simulink model "controller_archive2"  (R2022b)
settings: Solver=ode4  StartTime=0.0  StopTime=4  FixedStep=0.001  RelTol=1e-3
PreLoadFcn:
  | global m1 m2 l g m1_hat m2_hat;
  | m1 = 2;
  | m2 = 2;
  | m1_hat = 0.97*m1;
  | m2_hat = 0.97*m2;
  | l = 1;
  | g = 9.81;
  | 
  | kd = 200;
  | md = m1_hat;
  | dd = 2*0.7*sqrt(kd*md);
  | 
  | Kd = [kd,0;0,kd];
  | Md = [md,0;0,md];
  | Dd = [dd,0;0,dd];
  | 
  | p = 10^6;
  | d = 2*0.7*sqrt(p);
  | 
  | P = [p,0;0,p];
  | D = [d,0;0,d];
  | 
  | D_hold = D;
  | P_hold = P;
  | 
  | ke = 300;
  | Ke = [ke,0;0,0];
  | 
  | Fc = 1;
  | cv = 4;
  | 
  | delta = 0.01;
  | 
  | x0 = [0.95,0.95];
  | dx0 = [0;0];
  | 
  | n_pow = 0.001;
  | 
  | wall = 0.8;
  | 
  | delay = 2;
libraries: simulink x18, bbblueBasicLib x7
(part 2 of 2)

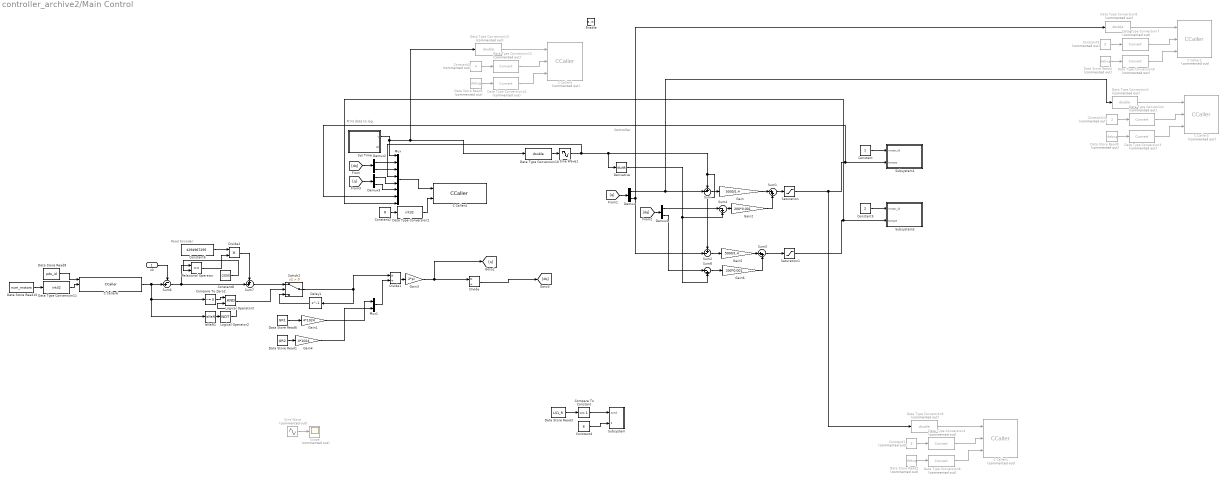
== system controller_archive2/Main Control ==
  note: Controller
  note: Print data to log
  note: Read Encoder
  x0 : Inport
  Enable : EnablePort
  C Caller1 : CCaller  Commented=on  FunctionName=print_input  PortSpecificationStruct="%)30     .    : 4   8    (     @         %    \"     ,    !     0         %  0 \"0    $    _    07)G3F%M90  4&]R=$YA;64 4V-O<&4     26YD97@     5'EP90      4VEZ90      27-';&]B86P   X    P    !@    @    $          4    (     0    $    !         !   0!A    #@   #     &    \"     0         !0    @    !     0    $         $  ! &$    .    .     8    (    !          %    \"     $    %     0         0    !0   $EN<'5T    #@   #@    &    \"     8         !0    @    !     0    $         \"0    @               X    X    !@    @    $          4    (     0    8    !         !     &    9&]U8FQE   .    ,     8    (    !          %    \"     $    !     0         0  $ ,0    X    P    !@    @    ) @        4    (     0    $    !          (  0      #@   #     &    \"     0         !0    @    !     @    $         $  \" &ED   .    ,     8    (    !          %    \"     $    \"     0         0  ( :60   X    X    !@    @    $          4    (     0    4    !         !     %    26YP=70    .    .     8    (    !@         %    \"     $    !     0         )    \"            / _#@   #@    &    \"     0         !0    @    !    !0    $         $     4   !I;G0S,@    X    P    !@    @    $          4    (     0    $    !         !   0 Q    #@   #     &    \"     D\"        !0    @    !     0    $          @ !       .    .     8    (    !          %    \"     $    %     0         0    !0   &1E8G5G    #@   #@    &    \"     0         !0    @    !    !0    $         $     4   !D96)U9P    X    X    !@    @    $          4    (     0    4    !         !     %    26YP=70    .    .     8    (    !@         %    \"     $    !     0         )    \"             ! #@   #@    &    \"     0         !0    @    !    !0    $         $     4   !I;G0S,@    X    P    !@    @    $          4    (     0    $    !         !   0 Q    #@   #     &    \"     D\"        !0    @    !     0    $          @ !"  SampleTime=0.001
  C Caller2 : CCaller  Commented=on  FunctionName=print_input  PortSpecificationStruct="%)30     .    : 4   8    (     @         %    \"     ,    !     0         %  0 \"0    $    _    07)G3F%M90  4&]R=$YA;64 4V-O<&4     26YD97@     5'EP90      4VEZ90      27-';&]B86P   X    P    !@    @    $          4    (     0    $    !         !   0!A    #@   #     &    \"     0         !0    @    !     0    $         $  ! &$    .    .     8    (    !          %    \"     $    %     0         0    !0   $EN<'5T    #@   #@    &    \"     8         !0    @    !     0    $         \"0    @               X    X    !@    @    $          4    (     0    8    !         !     &    9&]U8FQE   .    ,     8    (    !          %    \"     $    !     0         0  $ ,0    X    P    !@    @    ) @        4    (     0    $    !          (  0      #@   #     &    \"     0         !0    @    !     @    $         $  \" &ED   .    ,     8    (    !          %    \"     $    \"     0         0  ( :60   X    X    !@    @    $          4    (     0    4    !         !     %    26YP=70    .    .     8    (    !@         %    \"     $    !     0         )    \"            / _#@   #@    &    \"     0         !0    @    !    !0    $         $     4   !I;G0S,@    X    P    !@    @    $          4    (     0    $    !         !   0 Q    #@   #     &    \"     D\"        !0    @    !     0    $          @ !       .    .     8    (    !          %    \"     $    %     0         0    !0   &1E8G5G    #@   #@    &    \"     0         !0    @    !    !0    $         $     4   !D96)U9P    X    X    !@    @    $          4    (     0    4    !         !     %    26YP=70    .    .     8    (    !@         %    \"     $    !     0         )    \"             ! #@   #@    &    \"     0         !0    @    !    !0    $         $     4   !I;G0S,@    X    P    !@    @    $          4    (     0    $    !         !   0 Q    #@   #     &    \"     D\"        !0    @    !     0    $          @ !"  SampleTime=0.01
  C Caller3 : CCaller  Commented=on  FunctionName=print_input  PortSpecificationStruct="%)30     .    : 4   8    (     @         %    \"     ,    !     0         %  0 \"0    $    _    07)G3F%M90  4&]R=$YA;64 4V-O<&4     26YD97@     5'EP90      4VEZ90      27-';&]B86P   X    P    !@    @    $          4    (     0    $    !         !   0!A    #@   #     &    \"     0         !0    @    !     0    $         $  ! &$    .    .     8    (    !          %    \"     $    %     0         0    !0   $EN<'5T    #@   #@    &    \"     8         !0    @    !     0    $         \"0    @               X    X    !@    @    $          4    (     0    8    !         !     &    9&]U8FQE   .    ,     8    (    !          %    \"     $    !     0         0  $ ,0    X    P    !@    @    ) @        4    (     0    $    !          (  0      #@   #     &    \"     0         !0    @    !     @    $         $  \" &ED   .    ,     8    (    !          %    \"     $    \"     0         0  ( :60   X    X    !@    @    $          4    (     0    4    !         !     %    26YP=70    .    .     8    (    !@         %    \"     $    !     0         )    \"            / _#@   #@    &    \"     0         !0    @    !    !0    $         $     4   !I;G0S,@    X    P    !@    @    $          4    (     0    $    !         !   0 Q    #@   #     &    \"     D\"        !0    @    !     0    $          @ !       .    .     8    (    !          %    \"     $    %     0         0    !0   &1E8G5G    #@   #@    &    \"     0         !0    @    !    !0    $         $     4   !D96)U9P    X    X    !@    @    $          4    (     0    4    !         !     %    26YP=70    .    .     8    (    !@         %    \"     $    !     0         )    \"             ! #@   #@    &    \"     0         !0    @    !    !0    $         $     4   !I;G0S,@    X    P    !@    @    $          4    (     0    $    !         !   0 Q    #@   #     &    \"     D\"        !0    @    !     0    $          @ !"  SampleTime=0.001
  C Caller4 : CCaller  FunctionName=print_data  PortSpecificationStruct="%)30     .    P ,   8    (     @         %    \"     (    !     0         %  0 \"0    $    _    07)G3F%M90  4&]R=$YA;64 4V-O<&4     26YD97@     5'EP90      4VEZ90      27-';&]B86P   X    P    !@    @    $          4    (     0    0    !         !  ! !D871A#@   #     &    \"     0         !0    @    !    !     $         $  $ &1A=&$.    0     8    (    !          %    \"     $    +     0         0    \"P   $EN<'5T3W5T<'5T       .    .     8    (    !@         %    \"     $    !     0         )    \"               #@   #@    &    \"     0         !0    @    !    !@    $         $     8   !D;W5B;&4   X    P    !@    @    $          4    (     0    (    !         !   @ M,0  #@   #     &    \"     D\"        !0    @    !     0    $          @ !       .    ,     8    (    !          %    \"     $    $     0         0  0 <VEZ90X    P    !@    @    $          4    (     0    0    !         !  ! !S:7IE#@   #@    &    \"     0         !0    @    !    !0    $         $     4   !);G!U=     X    X    !@    @    &          4    (     0    $    !          D    (            \\#\\.    .     8    (    !          %    \"     $    %     0         0    !0   &EN=#,R    #@   #     &    \"     0         !0    @    !     0    $         $  ! #$    .    ,     8    (    \"0(        %    \"     $    !     0         \"  $"  SampleTime=0.001
  C Caller5 : CCaller  Commented=on  FunctionName=print_input  PortSpecificationStruct="%)30     .    : 4   8    (     @         %    \"     ,    !     0         %  0 \"0    $    _    07)G3F%M90  4&]R=$YA;64 4V-O<&4     26YD97@     5'EP90      4VEZ90      27-';&]B86P   X    P    !@    @    $          4    (     0    $    !         !   0!A    #@   #     &    \"     0         !0    @    !     0    $         $  ! &$    .    .     8    (    !          %    \"     $    %     0         0    !0   $EN<'5T    #@   #@    &    \"     8         !0    @    !     0    $         \"0    @               X    X    !@    @    $          4    (     0    8    !         !     &    9&]U8FQE   .    ,     8    (    !          %    \"     $    !     0         0  $ ,0    X    P    !@    @    ) @        4    (     0    $    !          (  0      #@   #     &    \"     0         !0    @    !     @    $         $  \" &ED   .    ,     8    (    !          %    \"     $    \"     0         0  ( :60   X    X    !@    @    $          4    (     0    4    !         !     %    26YP=70    .    .     8    (    !@         %    \"     $    !     0         )    \"            / _#@   #@    &    \"     0         !0    @    !    !0    $         $     4   !I;G0S,@    X    P    !@    @    $          4    (     0    $    !         !   0 Q    #@   #     &    \"     D\"        !0    @    !     0    $          @ !       .    .     8    (    !          %    \"     $    %     0         0    !0   &1E8G5G    #@   #@    &    \"     0         !0    @    !    !0    $         $     4   !D96)U9P    X    X    !@    @    $          4    (     0    4    !         !     %    26YP=70    .    .     8    (    !@         %    \"     $    !     0         )    \"             ! #@   #@    &    \"     0         !0    @    !    !0    $         $     4   !I;G0S,@    X    P    !@    @    $          4    (     0    $    !         !   0 Q    #@   #     &    \"     D\"        !0    @    !     0    $          @ !"  SampleTime=0.01
  C Caller6 : CCaller  FunctionName=get_encoder  PortSpecificationStruct="%)30     .    < 4   8    (     @         %    \"     ,    !     0         %  0 \"0    $    _    07)G3F%M90  4&]R=$YA;64 4V-O<&4     26YD97@     5'EP90      4VEZ90      27-';&]B86P   X    X    !@    @    $          4    (     0    8    !         !     &    <&1O7VED   .    .     8    (    !          %    \"     $    &     0         0    !@   '!D;U]I9   #@   #@    &    \"     0         !0    @    !    !0    $         $     4   !);G!U=     X    X    !@    @    &          4    (     0    $    !          D    (               .    .     8    (    !          %    \"     $    %     0         0    !0   &EN=#,R    #@   #     &    \"     0         !0    @    !     0    $         $  ! #$    .    ,     8    (    \"0(        %    \"     $    !     0         \"  $       X    P    !@    @    $          4    (     0    0    !         !  ! !S:7IE#@   #     &    \"     0         !0    @    !    !     $         $  $ '-I>F4.    .     8    (    !          %    \"     $    %     0         0    !0   $EN<'5T    #@   #@    &    \"     8         !0    @    !     0    $         \"0    @           #P/PX    X    !@    @    $          4    (     0    4    !         !     %    :6YT,S(    .    ,     8    (    !          %    \"     $    !     0         0  $ ,0    X    P    !@    @    ) @        4    (     0    $    !          (  0      #@   #     &    \"     0         !0    @    !     P    $         $  # '!O<P .    ,     8    (    !          %    \"     $    #     0         0  , <&]S  X   !     !@    @    $          4    (     0    L    !         !     +    26YP=71/=71P=70       X    X    !@    @    &          4    (     0    $    !          D    (             $ .    .     8    (    !          %    \"     $    &     0         0    !@   &1O=6)L90  #@   #     &    \"     0         !0    @    !     0    $         $  ! #(    .    ,     8    (    \"0(        %    \"     $    !     0         \"  $"  SampleTime=0.001
  Compare To Constant : simulink/Logic and Bit Operations/Compare To Constant  relop===  const=1  OutDataTypeStr=boolean
  Compare To Zero2 : simulink/Logic and Bit Operations/Compare To Zero  relop=~=  OutDataTypeStr=boolean
  Constant : Constant
  Constant1 : Constant  Commented=on  Value=3
  Constant14 : Constant  Commented=on  Value=2
  Constant2 : Constant  Value=8
  Constant3 : Constant  Commented=on  Value=4
  Constant4 : Constant  Value=6
  Constant5 : Constant  Value=2
  Constant6 : Constant  Value=4294967295
  Constant8 : Constant  Value=-2000
  Constant9 : Constant  Commented=on  Value=3
  Data Store Read1 : DataStoreRead  DataStoreName=GR2  IndexOptions=Index vector (dialog)  Indices=1  OutputSizes=1
  Data Store Read10 : DataStoreRead  DataStoreName=num_motors  IndexOptions=Index vector (dialog)  Indices=1  OutputSizes=1
  Data Store Read{2,4..5,9} (4 alike) : DataStoreRead  Commented=on  DataStoreName=debug  IndexOptions=Index vector (dialog)  Indices=1  OutputSizes=1
  Data Store Read3 : DataStoreRead  DataStoreName=LS1_R  IndexOptions=Index vector (dialog)  Indices=1  OutputSizes=1
  Data Store Read6 : DataStoreRead  DataStoreName=GR1  IndexOptions=Index vector (dialog)  Indices=1  OutputSizes=1
  Data Store Read8 : DataStoreRead  DataStoreName=pdo_id  IndexOptions=Index vector (dialog)  Indices=1  OutputSizes=1
  Data Type Conversion{,3..4,6..7,9,12,14} (8 alike) : DataTypeConversion  Commented=on  SaturateOnIntegerOverflow=off  RndMeth=Floor
  Data Type Conversion{1,5,8,13} (4 alike) : DataTypeConversion  Commented=on  OutDataTypeStr=double  SaturateOnIntegerOverflow=off  RndMeth=Floor
  Data Type Conversion10 : DataTypeConversion  OutDataTypeStr=double  SaturateOnIntegerOverflow=off  RndMeth=Floor
  Data Type Conversion11 : DataTypeConversion  OutDataTypeStr=int32  SaturateOnIntegerOverflow=off  RndMeth=Floor
  Data Type Conversion2 : DataTypeConversion  OutDataTypeStr=int32  SaturateOnIntegerOverflow=off  RndMeth=Floor
  Delay1 : Delay  DelayLength=1  InitialCondition=0
  Demux{,1..3} (4 alike) : Demux  Outputs=2
  Derivative : Derivative
  Divide : Product  Inputs=*/
  Divide1 : Product  Inputs=*/
  Divide2 : Product  Inputs=**
  Gain : Gain  Gain=5000/1.4
  Gain1 : Gain  Gain=4*1024
  Gain2 : Gain  Gain=200*0.001
  Gain3 : Gain  Gain=2*pi
  Gain4 : Gain  Gain=4*1024
  Gain5 : Gain  Gain=5000/1.4
  Gain6 : Gain  Gain=200*0.001
  IsNaN1 : RelationalOperator  Operator=isNaN  OutDataTypeStr=boolean  RndMeth=Simplest  InputSameDT=off
  Logical Operator2 : Logic  Operator=NOT  AllPortsSameDT=off  OutDataTypeStr=boolean
  Logical Operator3 : Logic  AllPortsSameDT=off  OutDataTypeStr=boolean
  Mux : Mux  Inputs=8
  Mux1 : Mux  Inputs=2
  Relational Operator : RelationalOperator  Operator=<=  OutDataTypeStr=boolean  RndMeth=Simplest  InputSameDT=off
  Saturation : Saturate  UpperLimit=400  LowerLimit=-400
  Saturation1 : Saturate  UpperLimit=400  LowerLimit=-400
  Scope : Scope  Commented=on
  Sine Wave : Sin  Commented=on  Amplitude=0.3  Bias=0.5  Frequency=0.1  SampleTime=0
  Sine Wave1 : Sin  TimeSource=Use external signal  Amplitude=0.3  Bias=0.3  Frequency=1.5  Phase=-pi/2  SampleTime=0
  Subsystem : Subsystem
  Subsystem1 : Subsystem
  Subsystem2 : Subsystem
  Sum : Sum  Inputs=+-|
  Sum1 : Sum  Inputs=|++
  Sum2 : Sum  Inputs=+-|
  Sum3 : Sum  Inputs=|++
  Sum4 : Sum  Inputs=|-+
  Sum6 : Sum  Inputs=-+|
  Sum7 : Sum  Inputs=++|
  Sum8 : Sum  Inputs=|-+
  Switch2 : Switch  Criteria=u2 > Threshold  SaturateOnIntegerOverflow=off  InputSameDT=off
  Sys Time : Subsystem
  wires:
  Constant/1 -> Subsystem1/1(motor_id)
  Constant2/1 -> Data Type Conversion2/1
  Mux/1 -> C Caller4/1
  Sys Time/1(t) -> Mux/1, Data Type Conversion13/1, Data Type Conversion10/1
  Data Type Conversion2/1 -> C Caller4/2
  [dq] -> Demux2/1
  Compare To Constant/1 -> Subsystem/1(cond)
  Constant4/1 -> Subsystem/2(new_state)
  Data Store Read3/1 -> Compare To Constant/1
  Constant14/1 -> Data Type Conversion/1
  Data Type Conversion3/1 -> C Caller3/3
  Data Store Read9/1 -> Data Type Conversion3/1
  Data Type Conversion/1 -> C Caller3/2
  Data Type Conversion1/1 -> C Caller3/1
  Data Store Read10/1 -> Data Type Conversion11/1
  Compare To Zero2/1 -> Logical Operator3/1
  Logical Operator2/1 -> Logical Operator3/2
  Delay1/1 -> Switch2/3
  IsNaN1/1 -> Logical Operator2/1
  Divide1/1 -> Gain3/1
  Logical Operator3/1 -> Switch2/2
  Data Store Read6/1 -> Gain1/1
  Gain1/1 -> Mux1/1
  Gain3/1 -> Divide/1, [q]
  Data Store Read8/1 -> C Caller6/1
  Divide/1 -> [dq]
  Data Type Conversion11/1 -> C Caller6/2
  x0/1 -> Sum6/1
  Sum6/1 -> Relational Operator/1, Sum7/2
  Constant6/1 -> Divide2/1
  Divide2/1 -> Sum7/1
  Sum7/1 -> Switch2/1
  Saturation/1 -> Data Type Conversion5/1, Mux/7, Subsystem1/2(torque)
  Sum/1 -> Gain/1
  Gain/1 -> Sum1/1
  [dq] -> Demux1/1
  Demux1/1 -> Sum4/1
  Sum1/1 -> Saturation/1
  [q] -> Demux/1
  Mux1/1 -> Divide1/2
  Data Store Read1/1 -> Gain4/1
  Gain4/1 -> Mux1/2
  Data Type Conversion5/1 -> C Caller1/1
  Data Type Conversion4/1 -> C Caller1/2
  Constant1/1 -> Data Type Conversion4/1
  Data Store Read2/1 -> Data Type Conversion6/1
  Data Type Conversion6/1 -> C Caller1/3
  Constant5/1 -> Subsystem2/1(motor_id)
  Saturation1/1 -> Mux/8, Subsystem2/2(torque)
  Sum3/1 -> Saturation1/1
  Gain6/1 -> Sum3/2
  Gain5/1 -> Sum3/1
  Demux/2 -> Sum2/2, Data Type Conversion8/1
  Sum2/1 -> Gain5/1
  Switch2/1 -> Divide1/1, Delay1/1
  Relational Operator/1 -> Divide2/2
  Constant8/1 -> Relational Operator/2
  C Caller6/1 -> IsNaN1/1, Compare To Zero2/1, Sum6/2
  Sine Wave/1 -> Scope/1
  Sum4/1 -> Gain2/1
  Sine Wave1/1 -> Mux/4, Sum2/1, Sum/1, Derivative/1
  Data Type Conversion8/1 -> C Caller2/1
  Data Type Conversion7/1 -> C Caller2/2
  Data Store Read4/1 -> Data Type Conversion9/1
  Constant9/1 -> Data Type Conversion7/1
  Data Type Conversion9/1 -> C Caller2/3
  Data Type Conversion10/1 -> Sine Wave1/1
  Gain2/1 -> Sum1/2
  Sum8/1 -> Gain6/1
  Derivative/1 -> Sum8/2, Sum4/2
  Demux1/2 -> Sum8/1
  Demux2/1 -> Mux/2
  Demux2/2 -> Mux/3
  Demux/1 -> Data Type Conversion1/1, Sum/2
  Data Type Conversion14/1 -> C Caller5/3
  Data Store Read5/1 -> Data Type Conversion14/1
  Data Type Conversion12/1 -> C Caller5/2
  Constant3/1 -> Data Type Conversion12/1
  Data Type Conversion13/1 -> C Caller5/1
  Demux3/1 -> Mux/5
  Demux3/2 -> Mux/6
  [q] -> Demux3/1

== system controller_archive2/Home1/Stop Motor1 ==
  Trigger : TriggerPort  VariantControl=(inherit)
  C Caller4 : CCaller  FunctionName=stop_motor  PortSpecificationStruct="%)30     .    Z ,   8    (     @         %    \"     (    !     0         %  0 \"0    $    _    07)G3F%M90  4&]R=$YA;64 4V-O<&4     26YD97@     5'EP90      4VEZ90      27-';&]B86P   X    X    !@    @    $          4    (     0    8    !         !     &    <&1O7V9D   .    .     8    (    !          %    \"     $    &     0         0    !@   '!D;U]F9   #@   #@    &    \"     0         !0    @    !    !0    $         $     4   !);G!U=     X    X    !@    @    &          4    (     0    $    !          D    (               .    .     8    (    !          %    \"     $    %     0         0    !0   &EN=#,R    #@   #     &    \"     0         !0    @    !     0    $         $  ! #$    .    ,     8    (    \"0(        %    \"     $    !     0         \"  $       X   !     !@    @    $          4    (     0    H    !         !     *    ;G5M7VUO=&]R<P        X   !     !@    @    $          4    (     0    H    !         !     *    ;G5M7VUO=&]R<P        X    X    !@    @    $          4    (     0    4    !         !     %    26YP=70    .    .     8    (    !@         %    \"     $    !     0         )    \"            / _#@   #@    &    \"     0         !0    @    !    !0    $         $     4   !I;G0S,@    X    P    !@    @    $          4    (     0    $    !         !   0 Q    #@   #     &    \"     D\"        !0    @    !     0    $          @ !"
  Data Store Read1 : DataStoreRead  DataStoreName=pdo_id  IndexOptions=Index vector (dialog)  Indices=1  OutputSizes=1
  Data Store Read7 : DataStoreRead  DataStoreName=num_motors  IndexOptions=Index vector (dialog)  Indices=1  OutputSizes=1
  Data Type Conversion : DataTypeConversion  OutDataTypeStr=int32  SaturateOnIntegerOverflow=off  RndMeth=Floor
  wires:
  Data Store Read1/1 -> C Caller4/1
  Data Store Read7/1 -> Data Type Conversion/1
  Data Type Conversion/1 -> C Caller4/2

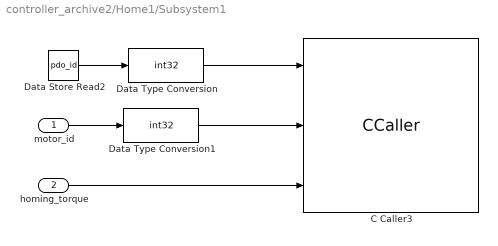
== system controller_archive2/Home1/Subsystem1 ==
  motor_id : Inport
  homing_torque : Inport  Port=2
  C Caller3 : CCaller  FunctionName=set_motor  PortSpecificationStruct="%)30     .    B 4   8    (     @         %    \"     ,    !     0         %  0 \"0    $    _    07)G3F%M90  4&]R=$YA;64 4V-O<&4     26YD97@     5'EP90      4VEZ90      27-';&]B86P   X    X    !@    @    $          4    (     0    8    !         !     &    <&1O7VED   .    .     8    (    !          %    \"     $    &     0         0    !@   '!D;U]I9   #@   #@    &    \"     0         !0    @    !    !0    $         $     4   !);G!U=     X    X    !@    @    &          4    (     0    $    !          D    (               .    .     8    (    !          %    \"     $    %     0         0    !0   &EN=#,R    #@   #     &    \"     0         !0    @    !     0    $         $  ! #$    .    ,     8    (    \"0(        %    \"     $    !     0         \"  $       X    X    !@    @    $          4    (     0    @    !         !     (    ;6]T;W)?:60.    .     8    (    !          %    \"     $    (     0         0    \"    &UO=&]R7VED#@   #@    &    \"     0         !0    @    !    !0    $         $     4   !);G!U=     X    X    !@    @    &          4    (     0    $    !          D    (            \\#\\.    .     8    (    !          %    \"     $    %     0         0    !0   &EN=#,R    #@   #     &    \"     0         !0    @    !     0    $         $  ! #$    .    ,     8    (    \"0(        %    \"     $    !     0         \"  $       X    X    !@    @    $          4    (     0    <    !         !     '    <V5T7W9A;  .    .     8    (    !          %    \"     $    '     0         0    !P   '-E=%]V86P #@   #@    &    \"     0         !0    @    !    !0    $         $     4   !);G!U=     X    X    !@    @    &          4    (     0    $    !          D    (             $ .    .     8    (    !          %    \"     $    &     0         0    !@   &1O=6)L90  #@   #     &    \"     0         !0    @    !     0    $         $  ! #$    .    ,     8    (    \"0(        %    \"     $    !     0         \"  $"  SampleTime=0.001
  Data Store Read2 : DataStoreRead  DataStoreName=pdo_id  IndexOptions=Index vector (dialog)  Indices=1  OutputSizes=1
  Data Type Conversion : DataTypeConversion  OutDataTypeStr=int32  SaturateOnIntegerOverflow=off  RndMeth=Floor
  Data Type Conversion1 : DataTypeConversion  OutDataTypeStr=int32  SaturateOnIntegerOverflow=off  RndMeth=Floor
  wires:
  motor_id/1 -> Data Type Conversion1/1
  Data Store Read2/1 -> Data Type Conversion/1
  Data Type Conversion/1 -> C Caller3/1
  Data Type Conversion1/1 -> C Caller3/2
  homing_torque/1 -> C Caller3/3

== system controller_archive2/Home1/Subsystem2 ==
  cond : Inport
  new_state : Inport  Port=2
  Data Store Read : DataStoreRead  DataStoreName=state  IndexOptions=Index vector (dialog)  Indices=1  OutputSizes=1
  Data Store Write : DataStoreWrite  DataStoreName=state  IndexOptions=Index vector (dialog)  Indices=1  OutputSizes=1
  Switch : Switch  Criteria=u2 > Threshold  SaturateOnIntegerOverflow=off  InputSameDT=off
  wires:
  new_state/1 -> Switch/1
  Data Store Read/1 -> Switch/3
  Switch/1 -> Data Store Write/1
  cond/1 -> Switch/2

== system controller_archive2/Home2/Stop Motor1 ==
  Trigger : TriggerPort  VariantControl=(inherit)
  C Caller4 : CCaller  FunctionName=stop_motor  PortSpecificationStruct="%)30     .    Z ,   8    (     @         %    \"     (    !     0         %  0 \"0    $    _    07)G3F%M90  4&]R=$YA;64 4V-O<&4     26YD97@     5'EP90      4VEZ90      27-';&]B86P   X    X    !@    @    $          4    (     0    8    !         !     &    <&1O7V9D   .    .     8    (    !          %    \"     $    &     0         0    !@   '!D;U]F9   #@   #@    &    \"     0         !0    @    !    !0    $         $     4   !);G!U=     X    X    !@    @    &          4    (     0    $    !          D    (               .    .     8    (    !          %    \"     $    %     0         0    !0   &EN=#,R    #@   #     &    \"     0         !0    @    !     0    $         $  ! #$    .    ,     8    (    \"0(        %    \"     $    !     0         \"  $       X   !     !@    @    $          4    (     0    H    !         !     *    ;G5M7VUO=&]R<P        X   !     !@    @    $          4    (     0    H    !         !     *    ;G5M7VUO=&]R<P        X    X    !@    @    $          4    (     0    4    !         !     %    26YP=70    .    .     8    (    !@         %    \"     $    !     0         )    \"            / _#@   #@    &    \"     0         !0    @    !    !0    $         $     4   !I;G0S,@    X    P    !@    @    $          4    (     0    $    !         !   0 Q    #@   #     &    \"     D\"        !0    @    !     0    $          @ !"
  Data Store Read1 : DataStoreRead  DataStoreName=pdo_id  IndexOptions=Index vector (dialog)  Indices=1  OutputSizes=1
  Data Store Read7 : DataStoreRead  DataStoreName=num_motors  IndexOptions=Index vector (dialog)  Indices=1  OutputSizes=1
  Data Type Conversion : DataTypeConversion  OutDataTypeStr=int32  SaturateOnIntegerOverflow=off  RndMeth=Floor
  wires:
  Data Store Read1/1 -> C Caller4/1
  Data Store Read7/1 -> Data Type Conversion/1
  Data Type Conversion/1 -> C Caller4/2

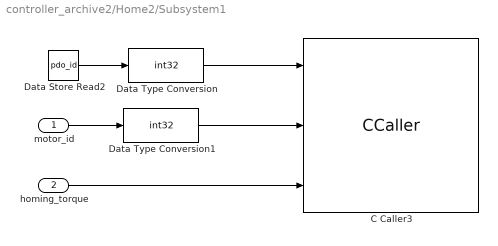
== system controller_archive2/Home2/Subsystem1 ==
  motor_id : Inport
  homing_torque : Inport  Port=2
  C Caller3 : CCaller  FunctionName=set_motor  PortSpecificationStruct="%)30     .    B 4   8    (     @         %    \"     ,    !     0         %  0 \"0    $    _    07)G3F%M90  4&]R=$YA;64 4V-O<&4     26YD97@     5'EP90      4VEZ90      27-';&]B86P   X    X    !@    @    $          4    (     0    8    !         !     &    <&1O7VED   .    .     8    (    !          %    \"     $    &     0         0    !@   '!D;U]I9   #@   #@    &    \"     0         !0    @    !    !0    $         $     4   !);G!U=     X    X    !@    @    &          4    (     0    $    !          D    (               .    .     8    (    !          %    \"     $    %     0         0    !0   &EN=#,R    #@   #     &    \"     0         !0    @    !     0    $         $  ! #$    .    ,     8    (    \"0(        %    \"     $    !     0         \"  $       X    X    !@    @    $          4    (     0    @    !         !     (    ;6]T;W)?:60.    .     8    (    !          %    \"     $    (     0         0    \"    &UO=&]R7VED#@   #@    &    \"     0         !0    @    !    !0    $         $     4   !);G!U=     X    X    !@    @    &          4    (     0    $    !          D    (            \\#\\.    .     8    (    !          %    \"     $    %     0         0    !0   &EN=#,R    #@   #     &    \"     0         !0    @    !     0    $         $  ! #$    .    ,     8    (    \"0(        %    \"     $    !     0         \"  $       X    X    !@    @    $          4    (     0    <    !         !     '    <V5T7W9A;  .    .     8    (    !          %    \"     $    '     0         0    !P   '-E=%]V86P #@   #@    &    \"     0         !0    @    !    !0    $         $     4   !);G!U=     X    X    !@    @    &          4    (     0    $    !          D    (             $ .    .     8    (    !          %    \"     $    &     0         0    !@   &1O=6)L90  #@   #     &    \"     0         !0    @    !     0    $         $  ! #$    .    ,     8    (    \"0(        %    \"     $    !     0         \"  $"  SampleTime=0.001
  Data Store Read2 : DataStoreRead  DataStoreName=pdo_id  IndexOptions=Index vector (dialog)  Indices=1  OutputSizes=1
  Data Type Conversion : DataTypeConversion  OutDataTypeStr=int32  SaturateOnIntegerOverflow=off  RndMeth=Floor
  Data Type Conversion1 : DataTypeConversion  OutDataTypeStr=int32  SaturateOnIntegerOverflow=off  RndMeth=Floor
  wires:
  motor_id/1 -> Data Type Conversion1/1
  Data Store Read2/1 -> Data Type Conversion/1
  Data Type Conversion/1 -> C Caller3/1
  Data Type Conversion1/1 -> C Caller3/2
  homing_torque/1 -> C Caller3/3

== system controller_archive2/Home2/Subsystem2 ==
  cond : Inport
  new_state : Inport  Port=2
  Data Store Read : DataStoreRead  DataStoreName=state  IndexOptions=Index vector (dialog)  Indices=1  OutputSizes=1
  Data Store Write : DataStoreWrite  DataStoreName=state  IndexOptions=Index vector (dialog)  Indices=1  OutputSizes=1
  Switch : Switch  Criteria=u2 > Threshold  SaturateOnIntegerOverflow=off  InputSameDT=off
  wires:
  new_state/1 -> Switch/1
  Data Store Read/1 -> Switch/3
  Switch/1 -> Data Store Write/1
  cond/1 -> Switch/2

== system controller_archive2/Home3/Stop Motor1 ==
  Trigger : TriggerPort  VariantControl=(inherit)
  C Caller4 : CCaller  FunctionName=stop_motor
  Data Store Read1 : DataStoreRead  DataStoreName=pdo_id  IndexOptions=Index vector (dialog)  Indices=1  OutputSizes=1
  Data Store Read7 : DataStoreRead  DataStoreName=num_motors  IndexOptions=Index vector (dialog)  Indices=1  OutputSizes=1
  Data Type Conversion : DataTypeConversion  OutDataTypeStr=int32  SaturateOnIntegerOverflow=off  RndMeth=Floor
  wires:
  Data Store Read1/1 -> C Caller4/1
  Data Store Read7/1 -> Data Type Conversion/1
  Data Type Conversion/1 -> C Caller4/2

== system controller_archive2/Home3/Subsystem1 ==
  motor_id : Inport
  homing_torque : Inport  Port=2
  C Caller3 : CCaller  FunctionName=set_motor  SampleTime=0.001
  Data Store Read2 : DataStoreRead  DataStoreName=pdo_id  IndexOptions=Index vector (dialog)  Indices=1  OutputSizes=1
  Data Type Conversion : DataTypeConversion  OutDataTypeStr=int32  SaturateOnIntegerOverflow=off  RndMeth=Floor
  Data Type Conversion1 : DataTypeConversion  OutDataTypeStr=int32  SaturateOnIntegerOverflow=off  RndMeth=Floor
  wires:
  motor_id/1 -> Data Type Conversion1/1
  Data Store Read2/1 -> Data Type Conversion/1
  Data Type Conversion/1 -> C Caller3/1
  Data Type Conversion1/1 -> C Caller3/2
  homing_torque/1 -> C Caller3/3

== system controller_archive2/Home3/Subsystem2 ==
  cond : Inport
  new_state : Inport  Port=2
  Data Store Read : DataStoreRead  DataStoreName=state  IndexOptions=Index vector (dialog)  Indices=1  OutputSizes=1
  Data Store Write : DataStoreWrite  DataStoreName=state  IndexOptions=Index vector (dialog)  Indices=1  OutputSizes=1
  Switch : Switch  Criteria=u2 > Threshold  SaturateOnIntegerOverflow=off  InputSameDT=off
  wires:
  new_state/1 -> Switch/1
  Data Store Read/1 -> Switch/3
  Switch/1 -> Data Store Write/1
  cond/1 -> Switch/2

== system controller_archive2/Home4/Stop Motor1 ==
  Trigger : TriggerPort  VariantControl=(inherit)
  C Caller4 : CCaller  FunctionName=stop_motor
  Data Store Read1 : DataStoreRead  DataStoreName=pdo_id  IndexOptions=Index vector (dialog)  Indices=1  OutputSizes=1
  Data Store Read7 : DataStoreRead  DataStoreName=num_motors  IndexOptions=Index vector (dialog)  Indices=1  OutputSizes=1
  Data Type Conversion : DataTypeConversion  OutDataTypeStr=int32  SaturateOnIntegerOverflow=off  RndMeth=Floor
  wires:
  Data Store Read1/1 -> C Caller4/1
  Data Store Read7/1 -> Data Type Conversion/1
  Data Type Conversion/1 -> C Caller4/2

== system controller_archive2/Home4/Subsystem1 ==
  motor_id : Inport
  homing_torque : Inport  Port=2
  C Caller3 : CCaller  FunctionName=set_motor  SampleTime=0.001
  Data Store Read2 : DataStoreRead  DataStoreName=pdo_id  IndexOptions=Index vector (dialog)  Indices=1  OutputSizes=1
  Data Type Conversion : DataTypeConversion  OutDataTypeStr=int32  SaturateOnIntegerOverflow=off  RndMeth=Floor
  Data Type Conversion1 : DataTypeConversion  OutDataTypeStr=int32  SaturateOnIntegerOverflow=off  RndMeth=Floor
  wires:
  motor_id/1 -> Data Type Conversion1/1
  Data Store Read2/1 -> Data Type Conversion/1
  Data Type Conversion/1 -> C Caller3/1
  Data Type Conversion1/1 -> C Caller3/2
  homing_torque/1 -> C Caller3/3

== system controller_archive2/Home4/Subsystem2 ==
  cond : Inport
  new_state : Inport  Port=2
  Data Store Read : DataStoreRead  DataStoreName=state  IndexOptions=Index vector (dialog)  Indices=1  OutputSizes=1
  Data Store Write : DataStoreWrite  DataStoreName=state  IndexOptions=Index vector (dialog)  Indices=1  OutputSizes=1
  Switch : Switch  Criteria=u2 > Threshold  SaturateOnIntegerOverflow=off  InputSameDT=off
  wires:
  new_state/1 -> Switch/1
  Data Store Read/1 -> Switch/3
  Switch/1 -> Data Store Write/1
  cond/1 -> Switch/2

== system controller_archive2/Initialize/Subsystem ==
  cond : Inport
  new_state : Inport  Port=2
  Data Store Read : DataStoreRead  DataStoreName=state  IndexOptions=Index vector (dialog)  Indices=1  OutputSizes=1
  Data Store Write : DataStoreWrite  DataStoreName=state  IndexOptions=Index vector (dialog)  Indices=1  OutputSizes=1
  Switch : Switch  Criteria=u2 > Threshold  SaturateOnIntegerOverflow=off  InputSameDT=off
  wires:
  new_state/1 -> Switch/1
  Data Store Read/1 -> Switch/3
  Switch/1 -> Data Store Write/1
  cond/1 -> Switch/2

== system controller_archive2/Main Control/Subsystem ==
  cond : Inport
  new_state : Inport  Port=2
  Data Store Read : DataStoreRead  DataStoreName=state  IndexOptions=Index vector (dialog)  Indices=1  OutputSizes=1
  Data Store Write : DataStoreWrite  DataStoreName=state  IndexOptions=Index vector (dialog)  Indices=1  OutputSizes=1
  Switch : Switch  Criteria=u2 > Threshold  SaturateOnIntegerOverflow=off  InputSameDT=off
  wires:
  new_state/1 -> Switch/1
  Data Store Read/1 -> Switch/3
  Switch/1 -> Data Store Write/1
  cond/1 -> Switch/2

== system controller_archive2/Main Control/Subsystem1 ==
  motor_id : Inport
  torque : Inport  Port=2
  C Caller3 : CCaller  FunctionName=set_motor  PortSpecificationStruct="%)30     .    B 4   8    (     @         %    \"     ,    !     0         %  0 \"0    $    _    07)G3F%M90  4&]R=$YA;64 4V-O<&4     26YD97@     5'EP90      4VEZ90      27-';&]B86P   X    X    !@    @    $          4    (     0    8    !         !     &    <&1O7VED   .    .     8    (    !          %    \"     $    &     0         0    !@   '!D;U]I9   #@   #@    &    \"     0         !0    @    !    !0    $         $     4   !);G!U=     X    X    !@    @    &          4    (     0    $    !          D    (               .    .     8    (    !          %    \"     $    %     0         0    !0   &EN=#,R    #@   #     &    \"     0         !0    @    !     0    $         $  ! #$    .    ,     8    (    \"0(        %    \"     $    !     0         \"  $       X    X    !@    @    $          4    (     0    @    !         !     (    ;6]T;W)?:60.    .     8    (    !          %    \"     $    (     0         0    \"    &UO=&]R7VED#@   #@    &    \"     0         !0    @    !    !0    $         $     4   !);G!U=     X    X    !@    @    &          4    (     0    $    !          D    (            \\#\\.    .     8    (    !          %    \"     $    %     0         0    !0   &EN=#,R    #@   #     &    \"     0         !0    @    !     0    $         $  ! #$    .    ,     8    (    \"0(        %    \"     $    !     0         \"  $       X    X    !@    @    $          4    (     0    <    !         !     '    <V5T7W9A;  .    .     8    (    !          %    \"     $    '     0         0    !P   '-E=%]V86P #@   #@    &    \"     0         !0    @    !    !0    $         $     4   !);G!U=     X    X    !@    @    &          4    (     0    $    !          D    (             $ .    .     8    (    !          %    \"     $    &     0         0    !@   &1O=6)L90  #@   #     &    \"     0         !0    @    !     0    $         $  ! #$    .    ,     8    (    \"0(        %    \"     $    !     0         \"  $"  SampleTime=0.001
  Data Store Read2 : DataStoreRead  DataStoreName=pdo_id  IndexOptions=Index vector (dialog)  Indices=1  OutputSizes=1
  Data Type Conversion : DataTypeConversion  OutDataTypeStr=int32  SaturateOnIntegerOverflow=off  RndMeth=Floor
  Data Type Conversion1 : DataTypeConversion  OutDataTypeStr=int32  SaturateOnIntegerOverflow=off  RndMeth=Floor
  wires:
  motor_id/1 -> Data Type Conversion1/1
  Data Store Read2/1 -> Data Type Conversion/1
  Data Type Conversion/1 -> C Caller3/1
  Data Type Conversion1/1 -> C Caller3/2
  torque/1 -> C Caller3/3

== system controller_archive2/Main Control/Subsystem2 ==
  motor_id : Inport
  torque : Inport  Port=2
  C Caller3 : CCaller  FunctionName=set_motor  PortSpecificationStruct="%)30     .    B 4   8    (     @         %    \"     ,    !     0         %  0 \"0    $    _    07)G3F%M90  4&]R=$YA;64 4V-O<&4     26YD97@     5'EP90      4VEZ90      27-';&]B86P   X    X    !@    @    $          4    (     0    8    !         !     &    <&1O7VED   .    .     8    (    !          %    \"     $    &     0         0    !@   '!D;U]I9   #@   #@    &    \"     0         !0    @    !    !0    $         $     4   !);G!U=     X    X    !@    @    &          4    (     0    $    !          D    (               .    .     8    (    !          %    \"     $    %     0         0    !0   &EN=#,R    #@   #     &    \"     0         !0    @    !     0    $         $  ! #$    .    ,     8    (    \"0(        %    \"     $    !     0         \"  $       X    X    !@    @    $          4    (     0    @    !         !     (    ;6]T;W)?:60.    .     8    (    !          %    \"     $    (     0         0    \"    &UO=&]R7VED#@   #@    &    \"     0         !0    @    !    !0    $         $     4   !);G!U=     X    X    !@    @    &          4    (     0    $    !          D    (            \\#\\.    .     8    (    !          %    \"     $    %     0         0    !0   &EN=#,R    #@   #     &    \"     0         !0    @    !     0    $         $  ! #$    .    ,     8    (    \"0(        %    \"     $    !     0         \"  $       X    X    !@    @    $          4    (     0    <    !         !     '    <V5T7W9A;  .    .     8    (    !          %    \"     $    '     0         0    !P   '-E=%]V86P #@   #@    &    \"     0         !0    @    !    !0    $         $     4   !);G!U=     X    X    !@    @    &          4    (     0    $    !          D    (             $ .    .     8    (    !          %    \"     $    &     0         0    !@   &1O=6)L90  #@   #     &    \"     0         !0    @    !     0    $         $  ! #$    .    ,     8    (    \"0(        %    \"     $    !     0         \"  $"  SampleTime=0.001
  Data Store Read2 : DataStoreRead  DataStoreName=pdo_id  IndexOptions=Index vector (dialog)  Indices=1  OutputSizes=1
  Data Type Conversion : DataTypeConversion  OutDataTypeStr=int32  SaturateOnIntegerOverflow=off  RndMeth=Floor
  Data Type Conversion1 : DataTypeConversion  OutDataTypeStr=int32  SaturateOnIntegerOverflow=off  RndMeth=Floor
  wires:
  motor_id/1 -> Data Type Conversion1/1
  Data Store Read2/1 -> Data Type Conversion/1
  Data Type Conversion/1 -> C Caller3/1
  Data Type Conversion1/1 -> C Caller3/2
  torque/1 -> C Caller3/3

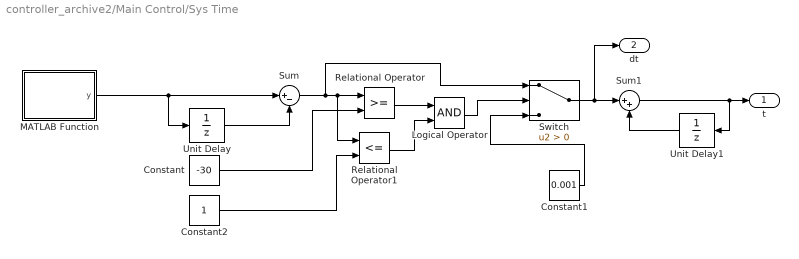
== system controller_archive2/Main Control/Sys Time ==
  Constant : Constant  Value=-30
  Constant1 : Constant  Value=0.001
  Constant2 : Constant
  Logical Operator : Logic  AllPortsSameDT=off  OutDataTypeStr=boolean
  MATLAB Function : MATLAB Function  TreatAsAtomicUnit=on
  Relational Operator : RelationalOperator  OutDataTypeStr=boolean  RndMeth=Simplest  InputSameDT=off
  Relational Operator1 : RelationalOperator  Operator=<=  OutDataTypeStr=boolean  RndMeth=Simplest  InputSameDT=off
  Sum : Sum  Inputs=|+-
  Sum1 : Sum  Inputs=|++
  Switch : Switch  Criteria=u2 > Threshold  SaturateOnIntegerOverflow=off  InputSameDT=off
  Unit Delay : UnitDelay  SampleTime=-1  HasFrameUpgradeWarning=on
  Unit Delay1 : UnitDelay  SampleTime=-1  HasFrameUpgradeWarning=on
  t : Outport
  dt : Outport  Port=2
  wires:
  MATLAB Function/1(y) -> Unit Delay/1, Sum/1
  Constant/1 -> Relational Operator/2
  Unit Delay1/1 -> Sum1/2
  Relational Operator1/1 -> Logical Operator/2
  Switch/1 -> dt/1, Sum1/1
  Sum/1 -> Relational Operator1/1, Relational Operator/1, Switch/1
  Sum1/1 -> t/1, Unit Delay1/1
  Unit Delay/1 -> Sum/2
  Relational Operator/1 -> Logical Operator/1
  Logical Operator/1 -> Switch/2
  Constant2/1 -> Relational Operator1/2
  Constant1/1 -> Switch/3

== matlab function controller_archive2/Main Control/Sys Time/MATLAB Function ==
  data: y output
function y = sysTime()
    c = datetime('now')
    y=c.Second;
